simulink model "MCU"  (R2024b)
settings: Solver=FixedStepAuto  StartTime=0.0  StopTime=5  FixedStep=5e-6  RelTol=1e-3
undefined symbols (not defined in the file): Ion, Lithium
libraries: canoelib x7, spsBatteryLib x1, spsPermanentMagnetSynchronousMachineLib x1, spsSeriesRLCBranchLib x1, spsUniversalBridgeLib x1, spspowerguiLib x1, slpidlib x1
settings Model: targetArch=x64  analysisModel=0  XcpMessageLength=-1  hasCAPLCallBlock=0  Creator=noname  LastModifiedBy=USER
settings SolverCC: AlgebraicLoopSolver=TrustRegion
settings DataIOCC: LimitDataPoints=on  SaveFormat=Array  ReturnWorkspaceOutputs=off
settings DebuggingCC: UnderspecifiedInitializationDetection=Classic  MergeDetectMultiDrivingBlocksExec=none  SolverPrmCheckMsg=warning  UnconnectedInputMsg=warning  UnconnectedOutputMsg=warning  UnconnectedLineMsg=warning  StateNameClashWarn=warning  SFUnexpectedBacktrackingDiag=warning  SFNoUnconditionalDefaultTransitionDiag=warning  SFExecutionAtInitializationDiag=none  ArithmeticOperatorsInVariantConditions=warning
settings ModelReferenceCC: EnableRefExpFcnMdlSchedulingChecks=on  PropagateSignalLabelsOutOfModel=off
settings SFSimCC: SimUseLocalCustomCode=off  CustomCodeUndefinedFunction=UseInterfaceOnly
settings RTWCC: Description=Vector CANoe Real-Time Target DLL (MinGW C/C++ Makefile)  SystemTargetFile=cn_mingw.tlc  TemplateMakefile=cn_mingw.tmf  RTWUseLocalCustomCode=off  GPUComputeCapability=3.5
settings CodeAppCC: StateflowObjectComments=on
settings STFCustomTargetCC: TargetLangStandard=C99 (ISO)  MatFileLogging=on  GRTInterface=on  SystemTargetFile=cn_mingw.tlc
settings GRTTargetCC: ParMdlRefBuildCompliant=off  CompOptLevelCompliant=off  ConcurrentExecutionCompliant=off  CombineOutputUpdateFcns=off  CPPClassGenCompliant=off  GRTInterface=on  UseToolchainInfoCompliant=off  RTWCAPISignals=on  RTWCAPIParams=on
settings ConfigComp: CovMetricSettings=dw  CovSaveCumulativeToWorkspaceVar=on  CovSaveSingleToWorkspaceVar=on  CovExternalEMLEnable=off
settings SimscapeCC: SimscapeNormalizeSystem=off

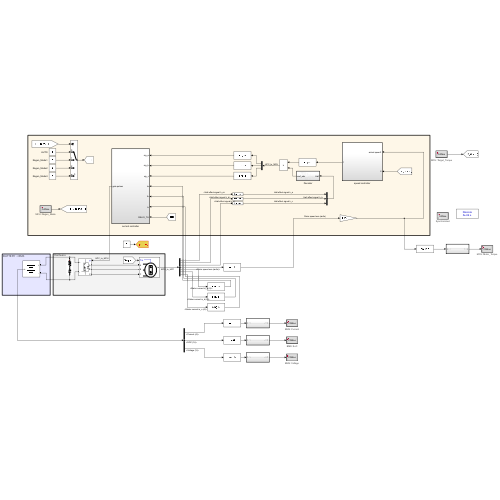
[thumbnail: Simulink's stored preview of the top-level diagram]
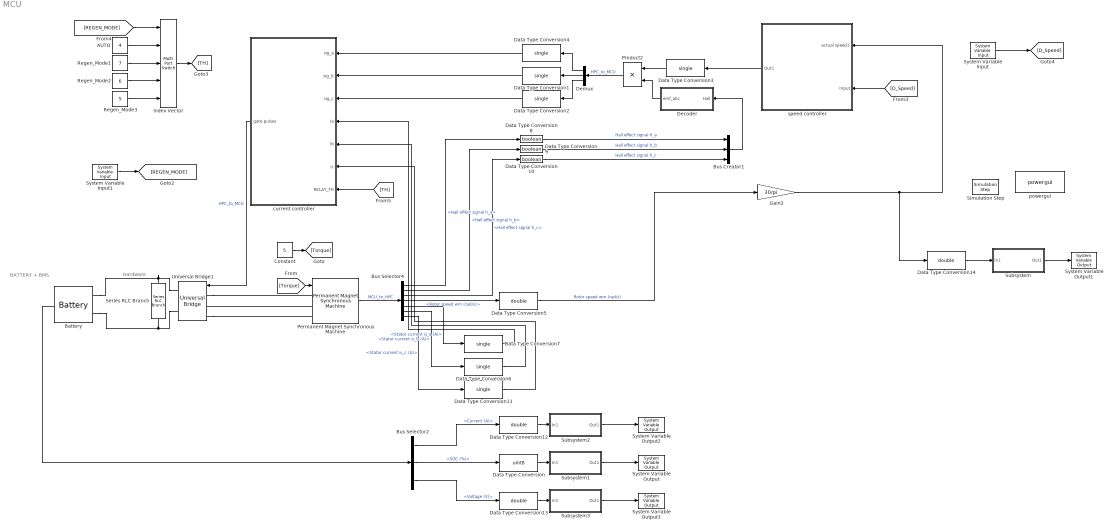
== system MCU ==
  note: BATTERY + BMS
  note: Hardware
  AUTO : Constant  Value=4
  Battery : spsBatteryLib/Battery  BatType=Lithium-Ion  NomV=48  NomQ=80  SOC=60  Batt_Tr=30  PresetModel=off  MaxQ=84  MinV=36  FullV=56.818272  Dis_rate=27.82608  R=0.006  Normal_OP=57.87524  expZone=[54.89208 3.144344]
      link override +: SampleTime=5e-6
      link override -: SampleTime=5e-6
      link override Controlled Voltage Source/+: SampleTime=5e-6
      link override Controlled Voltage Source/-: SampleTime=5e-6
      link override Controlled Voltage Source/s: SampleTime=5e-6
      link override Current Measurement/+: SampleTime=5e-6
      link override Current Measurement/-: SampleTime=5e-6
      link override Current Measurement/Model/in: SampleTime=5e-6
      link override Current Measurement/Model/out: SampleTime=5e-6
      link override Current Measurement/do not delete this gain: SampleTime=5e-6
      link override Current Measurement/i: SampleTime=5e-6
      link override Model/Discrete/Add: SampleTime=5e-6
      link override Model/Discrete/Compare To Zero/Compare: SampleTime=5e-6
      link override Model/Discrete/Compare To Zero/u: SampleTime=5e-6
      link override Model/Discrete/Compare To Zero/y: SampleTime=5e-6
      link override Model/Discrete/Compare To Zero1/Compare: SampleTime=5e-6
      link override Model/Discrete/Compare To Zero1/u: SampleTime=5e-6
      link override Model/Discrete/Compare To Zero1/y: SampleTime=5e-6
      link override Model/Discrete/Coulomb Counter: SampleTime=5e-6
      link override Model/Discrete/Current Filter: SampleTime=5e-6
      link override Model/Discrete/Data Type Conversion2: SampleTime=5e-6
      link override Model/Discrete/Exponential Zone Voltage/Abs: SampleTime=5e-6
      link override Model/Discrete/Exponential Zone Voltage/Add1: SampleTime=5e-6
      link override Model/Discrete/Exponential Zone Voltage/Cast To Double: SampleTime=5e-6
      link override Model/Discrete/Exponential Zone Voltage/Discrete-Time Integrator: SampleTime=5e-6
      link override Model/Discrete/Exponential Zone Voltage/Gain: SampleTime=5e-6
      link override Model/Discrete/Exponential Zone Voltage/Gain1: SampleTime=5e-6
      link override Model/Discrete/Exponential Zone Voltage/Product: SampleTime=5e-6
      link override Model/Discrete/Exponential Zone Voltage/Product1: SampleTime=5e-6
      link override Model/Discrete/Exponential Zone Voltage/current: SampleTime=5e-6
      link override Model/Discrete/Exponential Zone Voltage/exponentialZoneVoltage: SampleTime=5e-6
      link override Model/Discrete/Exponential Zone Voltage/isCharging: SampleTime=5e-6
      link override Model/Discrete/Gain: SampleTime=5e-6
      link override Model/Discrete/Gain1: SampleTime=5e-6
      link override Model/Discrete/Gain2: SampleTime=5e-6
      link override Model/Discrete/MATLAB Function/Capacity: SampleTime=5e-6
      link override Model/Discrete/MATLAB Function/CoulombCount: SampleTime=5e-6
      link override Model/Discrete/MATLAB Function/CoulombCountSaturated: SampleTime=5e-6
      link override Model/Discrete/MATLAB Function/CoulombCountSaturatedIntegrator: SampleTime=5e-6
      link override Model/Discrete/MATLAB Function/IsCharging: SampleTime=5e-6
      link override Model/Discrete/MATLAB Function/SaturatedConstant: SampleTime=5e-6
      link override Model/Discrete/Saturation: SampleTime=5e-6
      link override Model/Discrete/SoC/Fcn: SampleTime=5e-6
      link override Model/Discrete/SoC/Gain1: SampleTime=5e-6
      link override Model/Discrete/SoC/Saturation: SampleTime=5e-6
      link override Model/Discrete/SoC/SoC: SampleTime=5e-6
      link override Model/Discrete/SoC/capacity: SampleTime=5e-6
      link override Model/Discrete/SoC/coulombCount: SampleTime=5e-6
      link override Model/Discrete/Unit Delay: SampleTime=5e-6
      link override Model/Discrete/Voltage Loss Model/Lithium Ion/MATLAB Function/Capacity: SampleTime=5e-6
      link override Model/Discrete/Voltage Loss Model/Lithium Ion/MATLAB Function/ConstantA: SampleTime=5e-6
      link override Model/Discrete/Voltage Loss Model/Lithium Ion/MATLAB Function/ConstantB: SampleTime=5e-6
      link override Model/Discrete/Voltage Loss Model/Lithium Ion/MATLAB Function/ConstantK: SampleTime=5e-6
      link override Model/Discrete/Voltage Loss Model/Lithium Ion/MATLAB Function/CoulombCount: SampleTime=5e-6
      link override Model/Discrete/Voltage Loss Model/Lithium Ion/MATLAB Function/ExponentialZoneVoltage: SampleTime=5e-6
      link override Model/Discrete/Voltage Loss Model/Lithium Ion/MATLAB Function/FilteredCurrent: SampleTime=5e-6
      link override Model/Discrete/Voltage Loss Model/Lithium Ion/MATLAB Function/IsCharging: SampleTime=5e-6
      link override Model/Discrete/Voltage Loss Model/Lithium Ion/MATLAB Function/VoltageLoss: SampleTime=5e-6
      link override Model/Discrete/Voltage Loss Model/Lithium Ion/capacity: SampleTime=5e-6
      link override Model/Discrete/Voltage Loss Model/Lithium Ion/constantA: SampleTime=5e-6
      link override Model/Discrete/Voltage Loss Model/Lithium Ion/constantB: SampleTime=5e-6
      link override Model/Discrete/Voltage Loss Model/Lithium Ion/constantK: SampleTime=5e-6
      link override Model/Discrete/Voltage Loss Model/Lithium Ion/coulombCount: SampleTime=5e-6
      link override Model/Discrete/Voltage Loss Model/Lithium Ion/exponentialZoneVoltage: SampleTime=5e-6
      link override Model/Discrete/Voltage Loss Model/Lithium Ion/filteredCurrent: SampleTime=5e-6
      link override Model/Discrete/Voltage Loss Model/Lithium Ion/isCharging: SampleTime=5e-6
      link override Model/Discrete/Voltage Loss Model/Lithium Ion/voltageLoss: SampleTime=5e-6
      link override Model/Discrete/Voltage Loss Model/capacity: SampleTime=5e-6
      link override Model/Discrete/Voltage Loss Model/constantA: SampleTime=5e-6
      link override Model/Discrete/Voltage Loss Model/constantB: SampleTime=5e-6
      link override Model/Discrete/Voltage Loss Model/constantK: SampleTime=5e-6
      link override Model/Discrete/Voltage Loss Model/coulombCount: SampleTime=5e-6
      link override Model/Discrete/Voltage Loss Model/exponentialZoneVoltage: SampleTime=5e-6
      link override Model/Discrete/Voltage Loss Model/filteredCurrent: SampleTime=5e-6
      link override Model/Discrete/Voltage Loss Model/isCharging: SampleTime=5e-6
      link override Model/Discrete/Voltage Loss Model/voltageLoss: SampleTime=5e-6
      link override Model/Discrete/current: SampleTime=5e-6
      link override Model/Discrete/m: SampleTime=5e-6
      link override Model/Discrete/voltage: SampleTime=5e-6
      link override Model/current: SampleTime=5e-6
      link override Model/m: SampleTime=5e-6
      link override Model/voltage: SampleTime=5e-6
      link override m: SampleTime=5e-6
      settings: LibrarySourceBlock=electricdrivelib/Extra Sources/Battery
  Bus Creator1 : BusCreator  Inputs=3
  Bus Selector2 : BusSelector  OutputSignals=Current (A),SOC (%),Voltage (V)
  Bus Selector4 : BusSelector  OutputSignals=Hall effect signal h_a,Hall effect signal h_b,Hall effect signal h_c,Rotor speed wm (rad/s),Stator current is_a (A),Stator current is_b (A),Stator current is_c (A)
  Constant : Constant  Value=5
  Data Type Conversion : DataTypeConversion  OutDataTypeStr=uint8  SampleTime=5e-6  SaturateOnIntegerOverflow=off  RndMeth=Floor
  Data Type Conversion{1..4,6..7,11} (7 alike) : DataTypeConversion  OutDataTypeStr=single  SampleTime=5e-6  SaturateOnIntegerOverflow=off  RndMeth=Floor
  Data Type Conversion10 : DataTypeConversion  OutDataTypeStr=boolean  SampleTime=5e-6  SaturateOnIntegerOverflow=off  RndMeth=Floor
  Data Type Conversion{5,12..14} (4 alike) : DataTypeConversion  OutDataTypeStr=double  SampleTime=5e-6  SaturateOnIntegerOverflow=off  RndMeth=Floor
  Data Type Conversion8 : DataTypeConversion  OutDataTypeStr=boolean  SampleTime=5e-6  SaturateOnIntegerOverflow=off  RndMeth=Floor
  Data Type Conversion9 : DataTypeConversion  OutDataTypeStr=boolean  SampleTime=5e-6  SaturateOnIntegerOverflow=off  RndMeth=Floor
  Decoder : Subsystem  TreatAsAtomicUnit=on  SystemSampleTime=5e-6
  Demux : Demux  Outputs=3
  Gain2 : Gain  Gain=30/pi  SampleTime=5e-6
  Index Vector : MultiPortSwitch  DataPortOrder=Zero-based contiguous  Inputs=4  zeroidx=on  SampleTime=5e-6  SaturateOnIntegerOverflow=off  InputSameDT=off
  Permanent Magnet Synchronous Machine : spsPermanentMagnetSynchronousMachineLib/Permanent Magnet Synchronous Machine  NbPhases=3  FluxDistribution=Trapezoidal  RotorType=Round  MechanicalLoad=Torque Tm  PresetModel=No  ShowDetailedParameters=on  MeasurementBus=off  Resistance=0.0095  Inductance=0.0144e-3  dqInductances=[8.5e-3,8.5e-3]  La=0.000835  MachineConstant=Torque Constant (N.m / A_peak)  Flux=0.0059375  VoltageCst=9.9484  TorqueCst=0.095  Flat=120  Mechanical=[0.00019, 1e-6, 8, 0]  PolePairs=8  InitialConditions=[0,0, 0,0]  InitialConditions5ph=[0 0 0 0 0 0]  RefAngle=90 degrees behind phase A axis (modified Park)  IterativeDiscreteModel=Backward Euler robust  TsBlock=1e-3  TsPowergui=0
      link override A: SampleTime=5e-6
      link override B: SampleTime=5e-6
      link override C: SampleTime=5e-6
      link override Electrical model/-: SampleTime=1e-3
      link override "Electrical model/BEMF, Flux/E abc": SampleTime=5e-6
      link override "Electrical model/BEMF, Flux/Phase a/E": SampleTime=5e-6
      link override "Electrical model/BEMF, Flux/Phase a/Fcn": SampleTime=5e-6
      link override "Electrical model/BEMF, Flux/Phase a/Gain4": SampleTime=5e-6
      link override "Electrical model/BEMF, Flux/Phase a/Product1": SampleTime=5e-6
      link override "Electrical model/BEMF, Flux/Phase a/Saturation": SampleTime=5e-6
      link override "Electrical model/BEMF, Flux/Phase a/phi'r": SampleTime=5e-6
      link override "Electrical model/BEMF, Flux/Phase a/the,we": SampleTime=5e-6
      link override "Electrical model/BEMF, Flux/Phase b/E": SampleTime=5e-6
      link override "Electrical model/BEMF, Flux/Phase b/Fcn": SampleTime=5e-6
      link override "Electrical model/BEMF, Flux/Phase b/Gain4": SampleTime=5e-6
      link override "Electrical model/BEMF, Flux/Phase b/Product1": SampleTime=5e-6
      link override "Electrical model/BEMF, Flux/Phase b/Saturation": SampleTime=5e-6
      link override "Electrical model/BEMF, Flux/Phase b/phi'r": SampleTime=5e-6
      link override "Electrical model/BEMF, Flux/Phase b/the,we": SampleTime=5e-6
      link override "Electrical model/BEMF, Flux/Phase c/E": SampleTime=5e-6
      link override "Electrical model/BEMF, Flux/Phase c/Fcn": SampleTime=5e-6
      link override "Electrical model/BEMF, Flux/Phase c/Gain4": SampleTime=5e-6
      link override "Electrical model/BEMF, Flux/Phase c/Product1": SampleTime=5e-6
      link override "Electrical model/BEMF, Flux/Phase c/Saturation": SampleTime=5e-6
      link override "Electrical model/BEMF, Flux/Phase c/phi'r": SampleTime=5e-6
      link override "Electrical model/BEMF, Flux/Phase c/the,we": SampleTime=5e-6
      link override "Electrical model/BEMF, Flux/phi'r abc": SampleTime=5e-6
      link override "Electrical model/BEMF, Flux/the,we": SampleTime=5e-6
      link override Electrical model/Gain3: SampleTime=5e-6
      link override Electrical model/Hall effect sensor/Angle converter/Trigonometric Function: SampleTime=5e-6
      link override Electrical model/Hall effect sensor/Angle converter/Trigonometric Function2: SampleTime=5e-6
      link override Electrical model/Hall effect sensor/Angle converter/rad2deg: SampleTime=5e-6
      link override Electrical model/Hall effect sensor/Angle converter/the: SampleTime=5e-6
      link override Electrical model/Hall effect sensor/Angle converter/the_deg: SampleTime=5e-6
      link override Electrical model/Hall effect sensor/Data Type Conversion: SampleTime=5e-6
      link override Electrical model/Hall effect sensor/Data Type Conversion1: SampleTime=5e-6
      link override Electrical model/Hall effect sensor/Data Type Conversion2: SampleTime=5e-6
      link override Electrical model/Hall effect sensor/Hall: SampleTime=5e-6
      link override Electrical model/Hall effect sensor/Logical Operator: SampleTime=5e-6
      link override Electrical model/Hall effect sensor/Logical Operator1: SampleTime=5e-6
      link override Electrical model/Hall effect sensor/Logical Operator2: SampleTime=5e-6
      link override Electrical model/Hall effect sensor/Relational Operator1: SampleTime=5e-6
      link override Electrical model/Hall effect sensor/Relational Operator2: SampleTime=5e-6
      link override Electrical model/Hall effect sensor/Relational Operator3: SampleTime=5e-6
      link override Electrical model/Hall effect sensor/Relational Operator4: SampleTime=5e-6
      link override Electrical model/Hall effect sensor/Relational Operator5: SampleTime=5e-6
      link override Electrical model/Hall effect sensor/Relational Operator6: SampleTime=5e-6
      link override Electrical model/Hall effect sensor/the: SampleTime=5e-6
      link override Electrical model/Product: SampleTime=5e-6
      link override Electrical model/Selector: SampleTime=1e-3
      link override Electrical model/State equations/Eabc: SampleTime=1e-3
      link override Electrical model/State equations/State Ia/Eabc: SampleTime=1e-3
      link override Electrical model/State equations/State Ia/Fcn: SampleTime=1e-3
      link override Electrical model/State equations/State Ia/Gain2: SampleTime=1e-3
      link override Electrical model/State equations/State Ia/Vab,Vbc: SampleTime=1e-3
      link override Electrical model/State equations/State Ia/i: SampleTime=1e-3
      link override Electrical model/State equations/State Ib/Eabc: SampleTime=1e-3
      link override Electrical model/State equations/State Ib/Fcn: SampleTime=1e-3
      link override Electrical model/State equations/State Ib/Gain2: SampleTime=1e-3
      link override Electrical model/State equations/State Ib/Vab,Vbc: SampleTime=1e-3
      link override Electrical model/State equations/State Ib/i: SampleTime=1e-3
      link override Electrical model/State equations/Sum1: SampleTime=1e-3
      link override Electrical model/State equations/Vab,Vbc: SampleTime=1e-3
      link override Electrical model/State equations/is: SampleTime=1e-3
      link override Electrical model/Sum2: SampleTime=5e-6
      link override Electrical model/Te: SampleTime=5e-6
      link override Electrical model/i: SampleTime=5e-6
      link override Electrical model/m: SampleTime=5e-6
      link override Electrical model/the: SampleTime=5e-6
      link override Electrical model/v: SampleTime=5e-6
      link override Electrical model/we: SampleTime=5e-6
      link override Measurements/Out1: SampleTime=5e-6
      link override Measurements/m_e: SampleTime=5e-6
      link override Measurements/m_m: SampleTime=5e-6
      link override Mechanical model/Coulomb & Viscous Friction/Gain: SampleTime=5e-6
      link override Mechanical model/Coulomb & Viscous Friction/Gain1: SampleTime=5e-6
      link override Mechanical model/Coulomb & Viscous Friction/Sign: SampleTime=5e-6
      link override Mechanical model/Coulomb & Viscous Friction/Sum: SampleTime=5e-6
      link override Mechanical model/Coulomb & Viscous Friction/u: SampleTime=5e-6
      link override Mechanical model/Coulomb & Viscous Friction/y: SampleTime=5e-6
      link override Mechanical model/Fcn: SampleTime=5e-6
      link override Mechanical model/Gain: SampleTime=5e-6
      link override Mechanical model/Gain2: SampleTime=5e-6
      link override Mechanical model/Shaft: SampleTime=5e-6
      link override Mechanical model/Sum: SampleTime=5e-6
      link override Mechanical model/Te: SampleTime=5e-6
      link override Mechanical model/input: SampleTime=5e-6
      link override Mechanical model/m: SampleTime=5e-6
      link override Mechanical model/the: SampleTime=5e-6
      link override Mechanical model/we: SampleTime=5e-6
      link override m: SampleTime=5e-6
      link override mec: SampleTime=5e-6
  Product2 : Product  SaturateOnIntegerOverflow=on  SampleTime=5e-6  OutDataTypeStr=Inherit: Same as first input
  Regen_Mode1 : Constant  Value=7
  Regen_Mode2 : Constant  Value=6
  Regen_Mode3 : Constant  Value=5
  Series RLC Branch : spsSeriesRLCBranchLib/Series RLC Branch  LConnTagsString=__new0  RConnTagsString=__new0  BranchType=RC  Resistance=1e-2  Inductance=1e-3  SetiL0=off  InitialCurrent=0  Capacitance=75e-3  Setx0=off  InitialVoltage=0  Measurements=None
  Simulation Step : canoelib/CANoe I//O/Simulation Step  mode=Synchronized
      settings: AttributesFormatString=%<mode>  SourceProductName=Vector CANoe
  Subsystem : Subsystem  TreatAsAtomicUnit=on  SystemSampleTime=1e-2
  Subsystem1 : Subsystem  TreatAsAtomicUnit=on  SystemSampleTime=1e-2
  Subsystem2 : Subsystem  TreatAsAtomicUnit=on  SystemSampleTime=1e-2
  Subsystem3 : Subsystem  TreatAsAtomicUnit=on  SystemSampleTime=1e-2
  System Variable Input : canoelib/CANoe I//O/System Variable Input  nsName=MCU  sysVarName=Target_Torque  arrayIndex=-1  editSampleTime=0  rawValue=Default  dataType=Default  dataTypeDB=double  hasEncoding=off  dataTypeCANoe=Get from CANoe
      settings: AttributesFormatString=%<nsName>::%<sysVarName>  SourceProductName=Vector CANoe
  System Variable Input1 : canoelib/CANoe I//O/System Variable Input  nsName=MCU  sysVarName=Regen_Mode  arrayIndex=-1  editSampleTime=0  rawValue=Default  dataType=Default  dataTypeDB=uint32  hasEncoding=off  dataTypeCANoe=Get from CANoe
      settings: AttributesFormatString=%<nsName>::%<sysVarName>  SourceProductName=Vector CANoe
  System Variable Output : canoelib/CANoe I//O/System Variable Output  nsName=BMS  sysVarName=SoC  arrayIndex=-1  rawValue=Default  dataType=Default  dataTypeDB=double  hasEncoding=off  dataTypeCANoe=Get from CANoe
      settings: AttributesFormatString=%<nsName>::%<sysVarName>  SourceProductName=Vector CANoe
  System Variable Output1 : canoelib/CANoe I//O/System Variable Output  nsName=MCU  sysVarName=Motor_Torque  arrayIndex=-1  rawValue=Default  dataType=Default  dataTypeDB=double  hasEncoding=off  dataTypeCANoe=Get from CANoe
      settings: AttributesFormatString=%<nsName>::%<sysVarName>  SourceProductName=Vector CANoe
  System Variable Output2 : canoelib/CANoe I//O/System Variable Output  nsName=BMS  sysVarName=Current  arrayIndex=-1  rawValue=Default  dataType=Default  dataTypeDB=double  hasEncoding=off  dataTypeCANoe=Get from CANoe
      settings: AttributesFormatString=%<nsName>::%<sysVarName>  SourceProductName=Vector CANoe
  System Variable Output3 : canoelib/CANoe I//O/System Variable Output  nsName=BMS  sysVarName=Voltage  arrayIndex=-1  rawValue=Default  dataType=Default  dataTypeDB=double  hasEncoding=off  dataTypeCANoe=Get from CANoe
      settings: AttributesFormatString=%<nsName>::%<sysVarName>  SourceProductName=Vector CANoe
  Universal Bridge1 : spsUniversalBridgeLib/Universal Bridge  Arms=3  SnubberResistance=1e5  SnubberCapacitance=inf  Device=MOSFET / Diodes  Ron=1e-3  Lon=0  ForwardVoltages="[  0  0  ]"  ForwardVoltage=0  GTOparameters=[ 10e-6 , 20e-6 ]  IGBTparameters=[ 1e-6 , 2e-6 ]  Measurements=None  Measurements_2=None  converterType=Rectifier
      link override +: SampleTime=5e-6
      link override -: SampleTime=5e-6
      link override A: SampleTime=5e-6
      link override B: SampleTime=5e-6
      link override C: SampleTime=5e-6
      link override Model/Data Type Conversion: SampleTime=5e-6
      link override Model/Gate: SampleTime=5e-6
      link override Model/Uswitch: SampleTime=5e-6
      link override "Model/g1,d1,g2,d2, ...": SampleTime=5e-6
      link override Model/gate: SampleTime=5e-6
      link override Model/iSwitch: SampleTime=5e-6
      link override Model/itail: SampleTime=5e-6
      link override Model/m: SampleTime=5e-6
      link override Model/status: SampleTime=5e-6
      link override Model/vf: SampleTime=5e-6
      link override g: SampleTime=5e-6
  current controller : Subsystem  TreatAsAtomicUnit=on  SystemSampleTime=5e-6
  powergui : spspowerguiLib/powergui  Priority=2  SimulationMode=Discrete  SampleTime=5e-6  frequency=60  Iterations=50  frequencyindice=0  Pbase=100e6  ErrMax=1e-4  UnitsV=kV  UnitsW=MW  buscounter=0  FunctionMessages=off  echomessages=off  EnableUseOfTLC=off  CurrentSourceSwitches=off  DisableSnubberDevices=off  DisableRonSwitches=off  DisableVfSwitches=off  DisplayEquations=off  AutomaticDiscreteSolvers=off  SolverType=Tustin  Interpol=off  ExternalGateDelay=off  methode=off  Ts=0  x0status=blocks  SPID=off  SwTol=0  HookPort=off  NonlinearTolerance=1e-4  nMaxIteration=100  ContinueOnMaxIteration=off  RestoreLinks=warning  ResistiveCurrentMeasurement=off  Frange=[0:2:500]  Ylog=off  Xlog=on  ShowGrid=off  save=off  variable=ZData  structure=N  ZoomFFT=off  StartTime=0.0  cycles=1  DisplayStyle=1  fundamental=60  FreqAxis=off  MaxFrequency=1000  frequencyindicesteady=1  RmsSteady=1  display=off
  speed controller : Subsystem  TreatAsAtomicUnit=on  SystemSampleTime=5e-6
  wires:
  Bus Creator1/1 -> Decoder/1(Hall)
  Decoder/1(emf_abc) -> Product2/2
  Product2/1 -> Demux/1  "HPC_to_MCU"
  Data Type Conversion8/1 -> Bus Creator1/1  "Hall effect signal h_a"
  Data Type Conversion9/1 -> Bus Creator1/2  "Hall effect signal h_b"
  Data Type Conversion10/1 -> Bus Creator1/3  "Hall effect signal h_c"
  Demux/1 -> Data Type Conversion4/1
  Demux/2 -> Data Type Conversion1/1
  Demux/3 -> Data Type Conversion2/1
  speed controller/1(Out1) -> Data Type Conversion3/1
  Gain2/1 -> Data Type Conversion14/1, speed controller/1(actual speed1)
  [D_Speed] -> speed controller/2(Input)
  Data Type Conversion3/1 -> Product2/1
  Data Type Conversion5/1 -> Gain2/1  "Rotor speed wm (rad/s)"
  System Variable Input/1 -> [D_Speed]
  Bus Selector4/7 -> Data Type Conversion11/1  "<Stator current is_c (A)>"
  Data Type Conversion4/1 -> current controller/1(sig_a)
  Battery/1 -> Bus Selector2/1
  Data Type Conversion1/1 -> current controller/2(sig_b)
  current controller/1(gate pulses) -> Universal Bridge1/1  "HPC_to_MCU"
  Data Type Conversion7/1 -> current controller/4(Ia)
  Bus Selector4/2 -> Data Type Conversion9/1  "<Hall effect signal h_b>"
  Index Vector/1 -> [TH]
  Bus Selector4/3 -> Data Type Conversion10/1  "<Hall effect signal h_c>"
  Bus Selector4/1 -> Data Type Conversion8/1  "<Hall effect signal h_a>"
  Bus Selector2/2 -> Data Type Conversion/1  "<SOC (%)>"
  Bus Selector4/5 -> Data Type Conversion7/1  "<Stator current is_a (A)>"
  [REGEN_MODE] -> Index Vector/1
  Bus Selector4/4 -> Data Type Conversion5/1  "<Rotor speed wm (rad/s)>"
  Data Type Conversion2/1 -> current controller/3(sig_c)
  [Torque] -> Permanent Magnet Synchronous Machine/1
  Permanent Magnet Synchronous Machine/1 -> Bus Selector4/1  "MCU_to_HPC"
  Data Type Conversion6/1 -> current controller/5(Ib)
  [TH] -> current controller/7(RELAY_TH)
  AUTO/1 -> Index Vector/2
  Constant/1 -> [Torque]
  Regen_Mode3/1 -> Index Vector/5
  Bus Selector4/6 -> Data Type Conversion6/1  "<Stator current is_b (A)>"
  Regen_Mode2/1 -> Index Vector/4
  Regen_Mode1/1 -> Index Vector/3
  Data Type Conversion11/1 -> current controller/6(Ic)
  Subsystem/1(Out1) -> System Variable Output1/1
  Data Type Conversion/1 -> Subsystem1/1(In1)
  Subsystem1/1(Out1) -> System Variable Output/1
  Subsystem2/1(Out1) -> System Variable Output2/1
  Subsystem3/1(Out1) -> System Variable Output3/1
  Data Type Conversion13/1 -> Subsystem3/1(In1)
  Bus Selector2/1 -> Data Type Conversion12/1  "<Current (A)>"
  Bus Selector2/3 -> Data Type Conversion13/1  "<Voltage (V)>"
  Data Type Conversion12/1 -> Subsystem2/1(In1)
  Data Type Conversion14/1 -> Subsystem/1(In1)
  System Variable Input1/1 -> [REGEN_MODE]
  connections:
  Universal Bridge1/RConn2 -- Series RLC Branch/RConn1 -- Battery/LConn2
  Universal Bridge1/RConn1 -- Series RLC Branch/LConn1 -- Battery/LConn1
  Permanent Magnet Synchronous Machine/LConn2 -- Universal Bridge1/LConn2
  Universal Bridge1/LConn1 -- Permanent Magnet Synchronous Machine/LConn1
  Universal Bridge1/LConn3 -- Permanent Magnet Synchronous Machine/LConn3

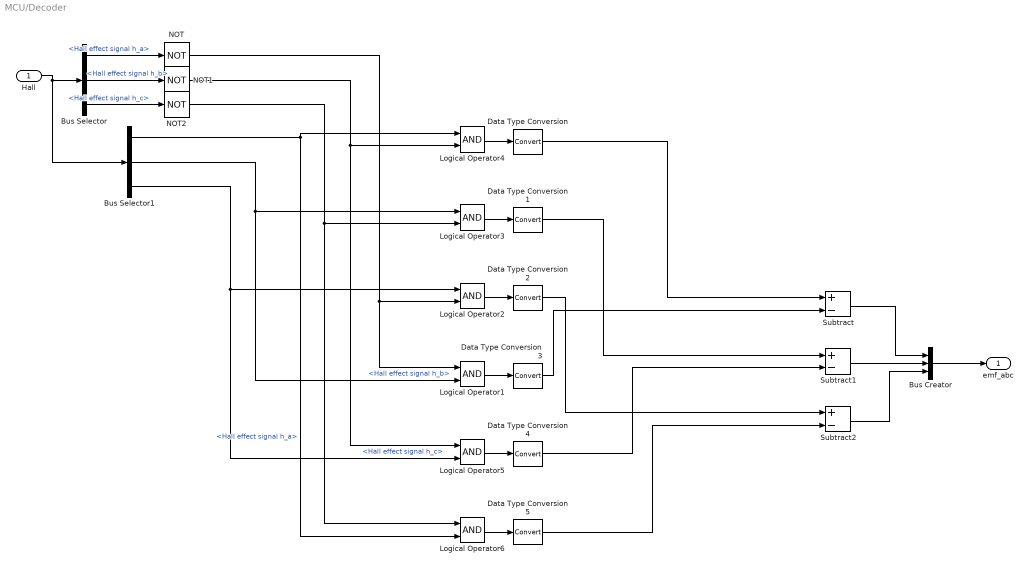
== system MCU/Decoder ==
  Hall : Inport  SampleTime=5e-6
  Bus Creator : BusCreator  Inputs=3
  Bus Selector : BusSelector  OutputSignals=Hall effect signal h_a,Hall effect signal h_b,Hall effect signal h_c
  Bus Selector1 : BusSelector  OutputSignals=Hall effect signal h_a,Hall effect signal h_b,Hall effect signal h_c
  Data Type Conversion{,1..5} (6 alike) : DataTypeConversion  SampleTime=5e-6
  Logical Operator{1..3,5..6} (5 alike) : Logic  AllPortsSameDT=off  SampleTime=5e-6
  Logical Operator4 : Logic  AllPortsSameDT=off  OutDataTypeStr=boolean  SampleTime=5e-6
  NOT : Logic  Operator=NOT  IconShape=distinctive  AllPortsSameDT=off  OutDataTypeStr=boolean  SampleTime=5e-6
  NOT1 : Logic  Operator=NOT  IconShape=distinctive  AllPortsSameDT=off  OutDataTypeStr=boolean  SampleTime=5e-6
  NOT2 : Logic  Operator=NOT  IconShape=distinctive  AllPortsSameDT=off  OutDataTypeStr=boolean  SampleTime=5e-6
  Subtract : Sum  Inputs=+-  SampleTime=5e-6
  Subtract1 : Sum  Inputs=+-  SampleTime=5e-6
  Subtract2 : Sum  Inputs=+-  SampleTime=5e-6
  emf_abc : Outport  SampleTime=5e-6
  wires:
  Bus Selector/3 -> NOT2/1  "<Hall effect signal h_c>"
  Logical Operator4/1 -> Data Type Conversion/1
  Logical Operator6/1 -> Data Type Conversion5/1
  Logical Operator2/1 -> Data Type Conversion2/1
  Logical Operator1/1 -> Data Type Conversion3/1
  Bus Selector1/3 -> Logical Operator5/2, Logical Operator2/1  "<Hall effect signal h_c>"
  Bus Selector1/1 -> Logical Operator4/1, Logical Operator6/2  "<Hall effect signal h_a>"
  Bus Selector/2 -> NOT1/1  "<Hall effect signal h_b>"
  Subtract/1 -> Bus Creator/1
  Subtract1/1 -> Bus Creator/2
  Data Type Conversion3/1 -> Subtract/2
  Subtract2/1 -> Bus Creator/3
  Data Type Conversion5/1 -> Subtract2/2
  Bus Selector1/2 -> Logical Operator3/1, Logical Operator1/2  "<Hall effect signal h_b>"
  Logical Operator5/1 -> Data Type Conversion4/1
  Data Type Conversion/1 -> Subtract/1
  Logical Operator3/1 -> Data Type Conversion1/1
  Bus Creator/1 -> emf_abc/1
  Data Type Conversion4/1 -> Subtract1/2
  Bus Selector/1 -> NOT/1  "<Hall effect signal h_a>"
  Data Type Conversion2/1 -> Subtract2/1
  Data Type Conversion1/1 -> Subtract1/1
  Hall/1 -> Bus Selector/1, Bus Selector1/1
  NOT/1 -> Logical Operator2/2, Logical Operator1/1
  NOT1/1 -> Logical Operator5/1, Logical Operator4/2
  NOT2/1 -> Logical Operator6/1, Logical Operator3/2

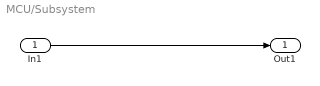
== system MCU/Subsystem ==
  In1 : Inport
  Out1 : Outport
  wires:
  In1/1 -> Out1/1

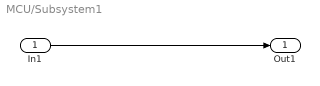
== system MCU/Subsystem1 ==
  In1 : Inport
  Out1 : Outport
  wires:
  In1/1 -> Out1/1

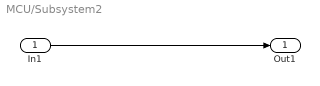
== system MCU/Subsystem2 ==
  In1 : Inport
  Out1 : Outport
  wires:
  In1/1 -> Out1/1

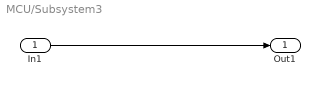
== system MCU/Subsystem3 ==
  In1 : Inport
  Out1 : Outport
  wires:
  In1/1 -> Out1/1

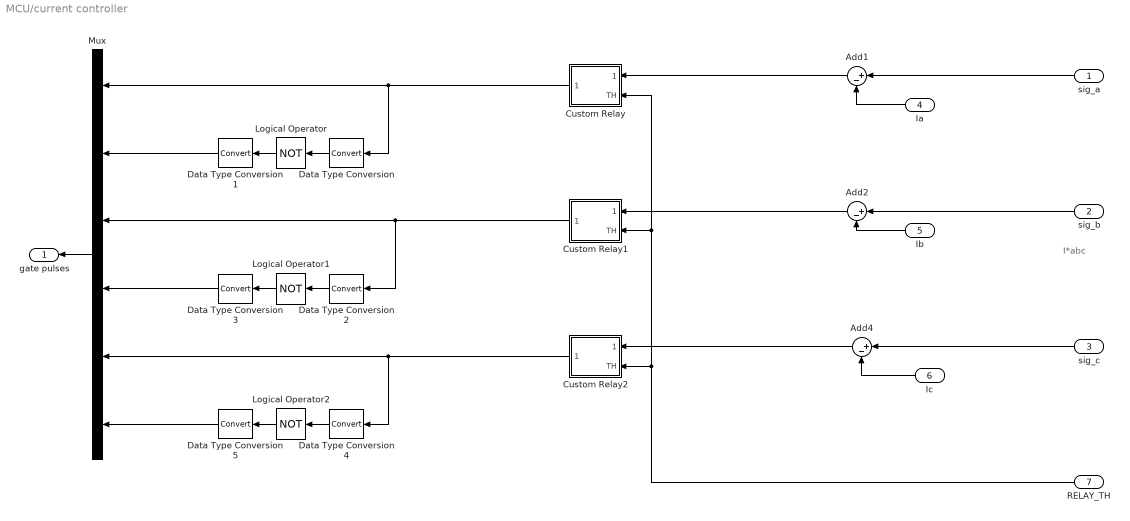
== system MCU/current controller ==
  note: I*abc
  sig_a : Inport  SampleTime=5e-6
  sig_b : Inport  Port=2  SampleTime=5e-6
  sig_c : Inport  Port=3  SampleTime=5e-6
  Ia : Inport  Port=4  SampleTime=5e-6
  Ib : Inport  Port=5  SampleTime=5e-6
  Ic : Inport  Port=6  SampleTime=5e-6
  RELAY_TH : Inport  Port=7  SampleTime=5e-6
  Add1 : Sum  Inputs=|+-  SampleTime=5e-6
  Add2 : Sum  Inputs=|+-  SampleTime=5e-6
  Add4 : Sum  Inputs=|+-  SampleTime=5e-6
  Custom Relay : Subsystem  TreatAsAtomicUnit=on  SystemSampleTime=5e-6
  Custom Relay1 : Subsystem  TreatAsAtomicUnit=on  SystemSampleTime=5e-6
  Custom Relay2 : Subsystem  TreatAsAtomicUnit=on  SystemSampleTime=5e-6
  Data Type Conversion{,1..5} (6 alike) : DataTypeConversion  SampleTime=5e-6
  Logical Operator : Logic  Operator=NOT  AllPortsSameDT=off  OutDataTypeStr=boolean  SampleTime=5e-6
  Logical Operator1 : Logic  Operator=NOT  AllPortsSameDT=off  OutDataTypeStr=boolean  SampleTime=5e-6
  Logical Operator2 : Logic  Operator=NOT  AllPortsSameDT=off  OutDataTypeStr=boolean  SampleTime=5e-6
  Mux : Mux  Inputs=6
  gate pulses : Outport  SampleTime=5e-6  VectorParamsAs1DForOutWhenUnconnected=off
  wires:
  Ib/1 -> Add2/2
  Mux/1 -> gate pulses/1
  Ic/1 -> Add4/2
  Add4/1 -> Custom Relay2/1(Signal)
  Add2/1 -> Custom Relay1/1(Signal)
  Add1/1 -> Custom Relay/1(Signal)
  Data Type Conversion/1 -> Logical Operator/1
  Logical Operator/1 -> Data Type Conversion1/1
  Data Type Conversion1/1 -> Mux/2
  Logical Operator1/1 -> Data Type Conversion3/1
  Data Type Conversion3/1 -> Mux/4
  Data Type Conversion2/1 -> Logical Operator1/1
  Data Type Conversion5/1 -> Mux/6
  Logical Operator2/1 -> Data Type Conversion5/1
  Data Type Conversion4/1 -> Logical Operator2/1
  sig_b/1 -> Add2/1
  sig_c/1 -> Add4/1
  Ia/1 -> Add1/2
  sig_a/1 -> Add1/1
  Custom Relay/1(Out1) -> Mux/1, Data Type Conversion/1
  Custom Relay1/1(Out1) -> Data Type Conversion2/1, Mux/3
  Custom Relay2/1(Out1) -> Data Type Conversion4/1, Mux/5
  RELAY_TH/1 -> Custom Relay2/2(TH), Custom Relay1/2(TH), Custom Relay/2(TH)

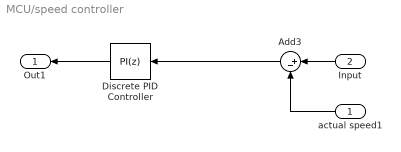
== system MCU/speed controller ==
  actual speed1 : Inport  SampleTime=5e-6
  Input : Inport  Port=2  SampleTime=5e-6
  Add3 : Sum  Inputs=|+-  OutDataTypeStr=double  SampleTime=5e-6
  Discrete PID Controller : slpidlib/PID Controller  Controller=PI  Form=Parallel  TimeDomain=Discrete-time  UseExternalTs=off  SampleTime=5e-6  IntegratorMethod=Forward Euler  FilterMethod=Forward Euler  ControllerParametersSource=internal  P=4.5  I=2.5  UseKiTs=off  D=0  UseExternalDerivativeSource=off  N=1  UseFilter=off  TunerSelectOption=Transfer Function Based (PID Tuner App)  InitialConditionSource=internal  InitialConditionForIntegrator=0  InitialConditionForFilter=0  DifferentiatorICPrevScaledInput=0  ExternalReset=none  TrackingMode=off  Kt=1  LimitOutput=off  SatLimitsSource=internal  UpperSaturationLimit=inf  LowerSaturationLimit=-inf  LinearizeAsGain=off  AntiWindupMode=none  Kb=1  LimitIntegrator=off  UpperIntegratorSaturationLimit=inf  LowerIntegratorSaturationLimit=-inf  POutMin=[]  POutMax=[]  IOutMin=[]  IOutMax=[]  DOutMin=[]  DOutMax=[]  NOutMin=[]  NOutMax=[]  SumOutMin=[]  SumOutMax=[]  SaturationOutMin=[]  SaturationOutMax=[]  PParamMin=[]  PParamMax=[]  IParamMin=[]  IParamMax=[]  DParamMin=[]  DParamMax=[]  NParamMin=[]  NParamMax=[]  KbParamMin=[]  KbParamMax=[]  KtParamMin=[]  KtParamMax=[]  KbOutMin=[]  KbOutMax=[]  KtOutMin=[]  KtOutMax=[]  IntegratorOutMin=[]  IntegratorOutMax=[]  FilterOutMin=[]  FilterOutMax=[]  SumI1OutMin=[]  SumI1OutMax=[]  SumI2OutMin=[]  SumI2OutMax=[]  SumI3OutMin=[]  SumI3OutMax=[]  SumI4OutMin=[]  SumI4OutMax=[]  SumDOutMin=[]  SumDOutMax=[]  DifferentiatorOutMin=[]  DifferentiatorOutMax=[]  FilterDiffOutCoefMin=[]  FilterDiffOutCoefMax=[]  ReciprocalOutMin=[]  ReciprocalOutMax=[]  SumDenOutMin=[]  SumDenOutMax=[]  SumNumOutMin=[]  SumNumOutMax=[]  DivideOutMin=[]  DivideOutMax=[]  UdiffTsProdOutMin=[]  UdiffTsProdOutMax=[]  NTsProdOutMin=[]  NTsProdOutMax=[]  UintegralTsProdOutMin=[]  UintegralTsProdOutMax=[]  UngainTsProdOutMin=[]  UngainTsProdOutMax=[]  ClampingZeroOutDataTypeStr=Inherit: Inherit via back propagation  ClampingZeroOutMin=[]  ClampingZeroOutMax=[]  FilterDenConstantOutDataTypeStr=Inherit: Inherit via back propagation  FilterDenConstantOutMin=[]  FilterDenConstantOutMax=[]  PCopyOutDataTypeStr=Inherit: Inherit via back propagation  PCopyOutMin=[]  PCopyOutMax=[]  NCopyOutDataTypeStr=Inherit: Inherit via back propagation  NCopyOutMin=[]  NCopyOutMax=[]  IntegratorContinuousStateAttributes=''  IntegratorStateMustResolveToSignalObject=off  IntegratorRTWStateStorageClass=Auto  FilterContinuousStateAttributes=''  FilterStateMustResolveToSignalObject=off  FilterRTWStateStorageClass=Auto  ParallelPVariant=InternalParameters  IdealPVariant=Disabled  IVariant=InternalParameters  DVariant=Disabled  IntegratorVariant=Discrete  SatVariant=Disabled  AWVariant=Passthrough  PCopyVariant=Disabled  TRVariant=Disabled  FdbkBlocksVariant=Forward  IdealPFdbkVariant=Disabled  SatFdbkVariant=Disabled  DerivativeFilterVariant=Disabled  NVariant=Disabled  NCopyVariant=Disabled_SignalSpec  FilterICVariant=Disabled  IntegratorICVariant=InternalICs  ExternalResetVariant=Disabled  TRSumVariant=Passthrough  SumFdbkVariant=Disabled  SumVariant=Sum_PI  TsampFilterVariant=InternalTs  TsampNgainVariant=Passthrough  TsampIntegralVariant=Disabled_SignalSpec  ExternalSaturationOutDataTypeStr=Inherit: Same as second input  DerivativeSourceVariant=Disabled  PreIntVariant=InternalPreInt
      link override D Gain/Internal Parameters/Derivative Gain: SampleTime=1e-3
      link override Filter/Disc. Forward Euler Filter/SumD: SampleTime=1e-3
      link override I Gain/Internal Parameters/Integral Gain: SampleTime=5e-6
      link override N Gain/Internal Parameters/Filter Coefficient: SampleTime=1e-3
      link override Parallel P Gain/Internal Parameters/Proportional Gain: SampleTime=5e-6
      link override Sum/Sum_PI/Sum: SampleTime=5e-6
      link override Sum/Sum_PID/Sum: SampleTime=1e-3
      link override Tracking Mode Sum/Passthrough/preInt: SampleTime=5e-6
      link override Tracking Mode Sum/preInt: SampleTime=5e-6
      settings: LibrarySourceBlock=simulink/Discrete/Discrete PID Controller
  Out1 : Outport  OutDataTypeStr=double  SampleTime=5e-6  VectorParamsAs1DForOutWhenUnconnected=off
  wires:
  Add3/1 -> Discrete PID Controller/1
  Discrete PID Controller/1 -> Out1/1
  actual speed1/1 -> Add3/2
  Input/1 -> Add3/1

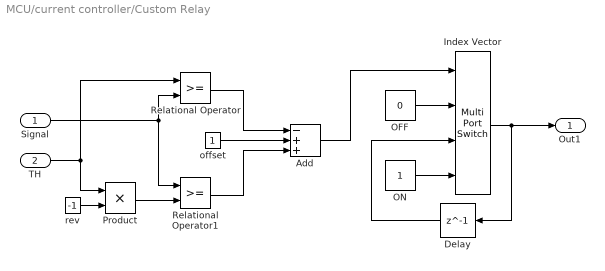
== system MCU/current controller/Custom Relay ==
  Signal : Inport  SampleTime=5e-6
  TH : Inport  Port=2  SampleTime=5e-6
  Add : Sum  Inputs=-++  SampleTime=5e-6
  Delay : Delay  DelayLength=1  InitialCondition=0  SampleTime=5e-6
  Index Vector : MultiPortSwitch  DataPortOrder=Zero-based contiguous  zeroidx=on  SampleTime=5e-6  SaturateOnIntegerOverflow=off  InputSameDT=off
  OFF : Constant  Value=0
  ON : Constant
  Product : Product  SampleTime=5e-6
  Relational Operator : RelationalOperator  OutDataTypeStr=boolean  SampleTime=5e-6  RndMeth=Simplest  InputSameDT=off
  Relational Operator1 : RelationalOperator  OutDataTypeStr=boolean  SampleTime=5e-6  RndMeth=Simplest  InputSameDT=off
  offset : Constant
  rev : Constant  Value=-1
  Out1 : Outport  SampleTime=5e-6
  wires:
  Relational Operator1/1 -> Add/3
  Relational Operator/1 -> Add/1
  Signal/1 -> Relational Operator1/1, Relational Operator/2
  Product/1 -> Relational Operator1/2
  TH/1 -> Relational Operator/1, Product/1
  offset/1 -> Add/2
  Add/1 -> Index Vector/1
  Index Vector/1 -> Delay/1, Out1/1
  ON/1 -> Index Vector/4
  OFF/1 -> Index Vector/2
  rev/1 -> Product/2
  Delay/1 -> Index Vector/3

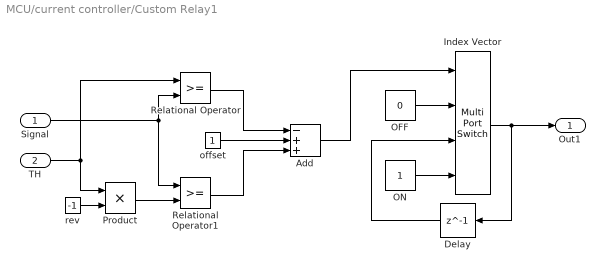
== system MCU/current controller/Custom Relay1 ==
  Signal : Inport  SampleTime=5e-6
  TH : Inport  Port=2  SampleTime=5e-6
  Add : Sum  Inputs=-++  SampleTime=5e-6
  Delay : Delay  DelayLength=1  InitialCondition=0  SampleTime=5e-6
  Index Vector : MultiPortSwitch  DataPortOrder=Zero-based contiguous  zeroidx=on  SampleTime=5e-6  SaturateOnIntegerOverflow=off  InputSameDT=off
  OFF : Constant  Value=0
  ON : Constant
  Product : Product  SampleTime=5e-6
  Relational Operator : RelationalOperator  OutDataTypeStr=boolean  SampleTime=5e-6  RndMeth=Simplest  InputSameDT=off
  Relational Operator1 : RelationalOperator  OutDataTypeStr=boolean  SampleTime=5e-6  RndMeth=Simplest  InputSameDT=off
  offset : Constant
  rev : Constant  Value=-1
  Out1 : Outport  SampleTime=5e-6
  wires:
  Relational Operator1/1 -> Add/3
  Relational Operator/1 -> Add/1
  Signal/1 -> Relational Operator1/1, Relational Operator/2
  Product/1 -> Relational Operator1/2
  TH/1 -> Relational Operator/1, Product/1
  offset/1 -> Add/2
  Add/1 -> Index Vector/1
  Index Vector/1 -> Delay/1, Out1/1
  ON/1 -> Index Vector/4
  OFF/1 -> Index Vector/2
  rev/1 -> Product/2
  Delay/1 -> Index Vector/3

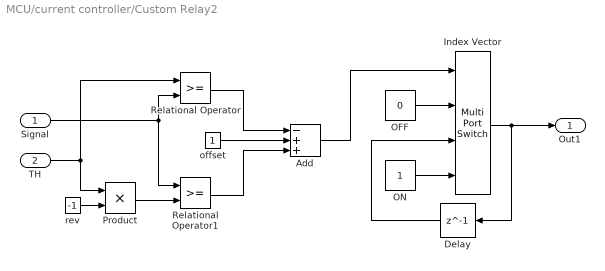
== system MCU/current controller/Custom Relay2 ==
  Signal : Inport  SampleTime=5e-6
  TH : Inport  Port=2  SampleTime=5e-6
  Add : Sum  Inputs=-++  SampleTime=5e-6
  Delay : Delay  DelayLength=1  InitialCondition=0  SampleTime=5e-6
  Index Vector : MultiPortSwitch  DataPortOrder=Zero-based contiguous  zeroidx=on  SampleTime=5e-6  SaturateOnIntegerOverflow=off  InputSameDT=off
  OFF : Constant  Value=0
  ON : Constant
  Product : Product  SampleTime=5e-6
  Relational Operator : RelationalOperator  OutDataTypeStr=boolean  SampleTime=5e-6  RndMeth=Simplest  InputSameDT=off
  Relational Operator1 : RelationalOperator  OutDataTypeStr=boolean  SampleTime=5e-6  RndMeth=Simplest  InputSameDT=off
  offset : Constant
  rev : Constant  Value=-1
  Out1 : Outport  SampleTime=5e-6
  wires:
  Relational Operator1/1 -> Add/3
  Relational Operator/1 -> Add/1
  Signal/1 -> Relational Operator1/1, Relational Operator/2
  Product/1 -> Relational Operator1/2
  TH/1 -> Relational Operator/1, Product/1
  offset/1 -> Add/2
  Add/1 -> Index Vector/1
  Index Vector/1 -> Delay/1, Out1/1
  ON/1 -> Index Vector/4
  OFF/1 -> Index Vector/2
  rev/1 -> Product/2
  Delay/1 -> Index Vector/3
